simulink model "DYNAMIC_SYSTEM"  (R2020b)
settings: Solver=VariableStepAuto  StartTime=0.0  StopTime=10  RelTol=1e-3
model workspace (MAT data in the model file):
  Sig = Simulink.Signal
  Sig.DataType = 'auto'
  Sig.Dimensions = -1
  Sig.DimensionsMode = 'auto'
  Sig.Complexity = 'auto'
  Sig.SampleTime = -1
  Sig.SamplingMode = 'auto'
  b = 50
  k1 = 50
  k12 = 50
  m1 = 100
  m2 = 100
  out = Simulink.SimulationOutput
  out.Data.tout = [0 0.000252982212813 0.000505964425627 0.00075894663844 0.00186292796113 0.00296690928383 0.00407089060652 0.00517487192921 0.00853265505613 0.0118904381831 0.01524822131 0.0186060044369 ... (2482 elements, 2482x1)]
  out.Metadata = Simulink.SimulationMetadata
  out.Metadata.ModelInfo.ModelName = 'DYNAMIC_SYSTEM'
  out.Metadata.ModelInfo.ModelVersion = '1.8'
  out.Metadata.ModelInfo.ModelFilePath = 'D:\KPIT\PROBLEM_1_DYNAMIC_SYSTEM\Simulink Model\DYNAMIC_SYSTEM.slx'
  out.Metadata.ModelInfo.UserID = 'intel'
  out.Metadata.ModelInfo.MachineName = 'DESKTOP-HTPAP2M'
  out.Metadata.ModelInfo.Platform = 'PCWIN64'
  out.Metadata.ModelInfo.ModelStructuralChecksum = [3337711430; 1140132305; 3994184035; 4274736616]
  out.Metadata.ModelInfo.SimulationMode = 'normal'
  out.Metadata.ModelInfo.StartTime = 0
  out.Metadata.ModelInfo.StopTime = 100
  out.Metadata.ModelInfo.SolverInfo.Type = 'Variable-Step'
  out.Metadata.ModelInfo.SolverInfo.Solver = 'ode15s'
  out.Metadata.ModelInfo.SolverInfo.MaxStepSize = 0.20964360587
  out.Metadata.ModelInfo.SimulinkVersion.Name = 'Simulink'
  out.Metadata.ModelInfo.SimulinkVersion.Version = '10.2'
  out.Metadata.ModelInfo.SimulinkVersion.Release = '(R2020b)'
  out.Metadata.ModelInfo.SimulinkVersion.Date = '29-Jul-2020'
  out.Metadata.ModelInfo.LoggingInfo.LoggingToFile = 'off'
  out.Metadata.TimingInfo.WallClockTimestampStart = '2020-12-05 15:58:28'
  out.Metadata.TimingInfo.WallClockTimestampStop = '2020-12-05 15:58:31'
  out.Metadata.TimingInfo.InitializationElapsedWallTime = 2.1436633
  out.Metadata.TimingInfo.ExecutionElapsedWallTime = 0.932311
  out.Metadata.TimingInfo.TerminationElapsedWallTime = 0.0153927
  out.Metadata.TimingInfo.TotalElapsedWallTime = 3.091367
  out.Metadata.TimingInfo.ProfilerData = 'Profiler is not enabled'
  out.Metadata.ExecutionInfo.StopEvent = 'ReachedStopTime'
  out.Metadata.ExecutionInfo.StopEventSource = []
  out.Metadata.ExecutionInfo.StopEventDescription = 'Reached stop time of 100'
  out.Metadata.ExecutionInfo.ErrorDiagnostic = []
  out.Metadata.ExecutionInfo.WarningDiagnostics = struct([])
  out.Metadata.AppInfo = struct()
libraries: pid_lib x1
settings Model: Creator=intel  LastModifiedBy=intel

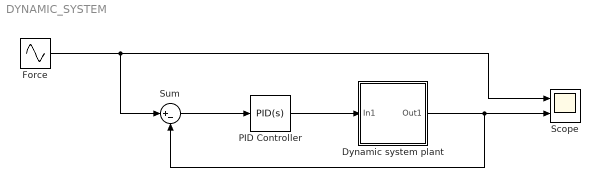
== system DYNAMIC_SYSTEM ==
  " PID Controller" : pid_lib/PID Controller  Controller=PID  Form=Parallel  TimeDomain=Continuous-time  UseExternalTs=off  SampleTime=-1  IntegratorMethod=Forward Euler  FilterMethod=Forward Euler  ControllerParametersSource=internal  P=1  I=1  D=0  UseFilter=on  N=100  TunerSelectOption=Transfer Function Based (PID Tuner App)  InitialConditionSource=internal  InitialConditionForIntegrator=0  InitialConditionForFilter=0  DifferentiatorICPrevScaledInput=0  ExternalReset=none  TrackingMode=off  Kt=1  LimitOutput=off  SatLimitsSource=internal  UpperSaturationLimit=inf  LowerSaturationLimit=-inf  LinearizeAsGain=on  AntiWindupMode=none  Kb=1  POutMin=[]  POutMax=[]  IOutMin=[]  IOutMax=[]  DOutMin=[]  DOutMax=[]  NOutMin=[]  NOutMax=[]  SumOutMin=[]  SumOutMax=[]  SaturationOutMin=[]  SaturationOutMax=[]  PParamMin=[]  PParamMax=[]  IParamMin=[]  IParamMax=[]  DParamMin=[]  DParamMax=[]  NParamMin=[]  NParamMax=[]  KbParamMin=[]  KbParamMax=[]  KtParamMin=[]  KtParamMax=[]  KbOutMin=[]  KbOutMax=[]  KtOutMin=[]  KtOutMax=[]  IntegratorOutMin=[]  IntegratorOutMax=[]  FilterOutMin=[]  FilterOutMax=[]  SumI1OutMin=[]  SumI1OutMax=[]  SumI2OutMin=[]  SumI2OutMax=[]  SumI3OutMin=[]  SumI3OutMax=[]  SumI4OutMin=[]  SumI4OutMax=[]  SumDOutMin=[]  SumDOutMax=[]  DifferentiatorOutMin=[]  DifferentiatorOutMax=[]  FilterDiffOutCoefMin=[]  FilterDiffOutCoefMax=[]  ReciprocalOutMin=[]  ReciprocalOutMax=[]  SumDenOutMin=[]  SumDenOutMax=[]  SumNumOutMin=[]  SumNumOutMax=[]  DivideOutMin=[]  DivideOutMax=[]  UdiffTsProdOutMin=[]  UdiffTsProdOutMax=[]  NTsProdOutMin=[]  NTsProdOutMax=[]  UintegralTsProdOutMin=[]  UintegralTsProdOutMax=[]  UngainTsProdOutMin=[]  UngainTsProdOutMax=[]  IntegratorContinuousStateAttributes=''  IntegratorStateMustResolveToSignalObject=off  IntegratorRTWStateStorageClass=Auto  FilterContinuousStateAttributes=''  FilterStateMustResolveToSignalObject=off  FilterRTWStateStorageClass=Auto  ParallelPVariant=InternalParameters  IdealPVariant=Disabled  IVariant=InternalParameters  DVariant=InternalParameters  IntegratorVariant=Continuous  SatVariant=Disabled  AWVariant=Passthrough  PCopyVariant=Disabled  TRVariant=Disabled  FdbkBlocksVariant=Forward  IdealPFdbkVariant=Disabled  SatFdbkVariant=Disabled  DerivativeFilterVariant=ContFilter  NVariant=InternalParameters  NCopyVariant=Disabled  FilterICVariant=InternalICsFilter  IntegratorICVariant=InternalICs  ExternalResetVariant=Disabled  TRSumVariant=Passthrough  SumFdbkVariant=Disabled  SumVariant=Sum_PID  TsampFilterVariant=InternalTs  TsampNgainVariant=Passthrough  TsampIntegralVariant=Passthrough  ExternalSaturationOutDataTypeStr=Inherit: Same as second input
  "Dynamic system plant " : Subsystem  mask{m2=100, k12=50}
      mask prompts: m2 "Mass(m2)"; k12 "Spring Constant(k12)"
  Force : Sin  Amplitude=2  Frequency=10  SampleTime=0
  Scope : Scope  NumInputPorts=2
  Sum : Sum  Inputs=|+-
  wires:
  Force/1 -> Sum/1, Scope/1
  "Dynamic system plant "/1(Out1) -> Scope/2, Sum/2
  Sum/1 -> " PID Controller"/1
  " PID Controller"/1 -> "Dynamic system plant "/1(In1)

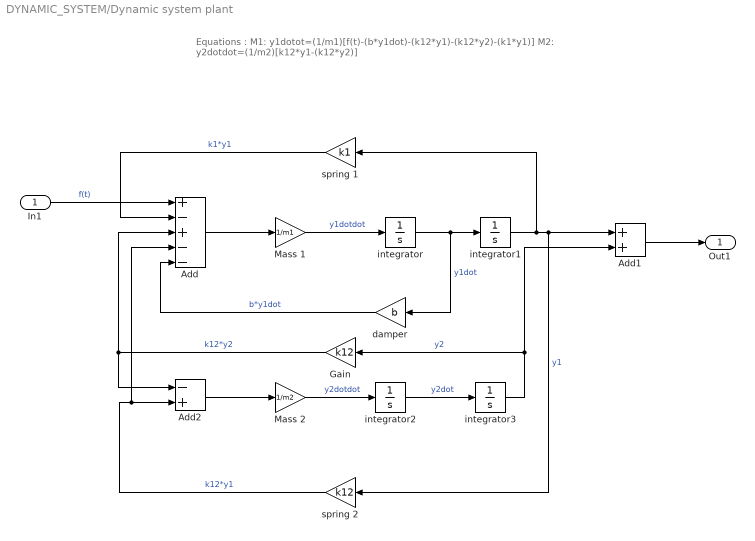
== system DYNAMIC_SYSTEM/Dynamic system plant  ==
  note: Equations :
      | M1:
      | y1dotot=(1/m1)[f(t)-(b*y1dot)-(k12*y1)-(k12*y2)-(k1*y1)]
      | M2:
      | y2dotdot=(1/m2)[k12*y1-(k12*y2)]
  In1 : Inport
  Add : Sum  Inputs=+-+--
  Add1 : Sum
  Add2 : Sum  Inputs=-+
  Gain : Gain  Gain=k12
  Mass 1 : Gain  Gain=1/m1
  Mass 2 : Gain  Gain=1/m2
  damper : Gain  Gain=b
  integrator{,1..3} (4 alike) : Integrator
  spring 1 : Gain  Gain=k1
  spring 2 : Gain  Gain=k12
  Out1 : Outport
  wires:
  Mass 2/1 -> integrator2/1  "y2dotdot"
  integrator/1 -> damper/1, integrator1/1  "y1dot"
  integrator1/1 -> spring 2/1, Add1/1, spring 1/1  "y1"
  Mass 1/1 -> integrator/1  "y1dotdot"
  spring 2/1 -> Add/4, Add2/2  "k12*y1"
  Add/1 -> Mass 1/1
  spring 1/1 -> Add/2  "k1*y1"
  integrator2/1 -> integrator3/1  "y2dot"
  damper/1 -> Add/5  "b*y1dot"
  In1/1 -> Add/1  "f(t)"
  Add1/1 -> Out1/1
  integrator3/1 -> Add1/2, Gain/1  "y2"
  Gain/1 -> Add/3, Add2/1  "k12*y2"
  Add2/1 -> Mass 2/1
